simulink model "GNC2026"  (R2024b)
settings: Solver=ode4  StartTime=0.0  StopTime=tsim  FixedStep=baseRate
values from neighbouring files (symbols this model uses):
  a = 1    [Run_Initializer.m]    (also in UKFoptimization.m)
  a1 = 0.236940    (= 0.23694)    [DrawARM.m]    (also in Run_Initializer.m = 2)
  a2 = 0.281536    [DrawARM.m]    (also in Run_Initializer.m = 2)
  a3 = 0.0621    [DrawARM.m]    (also in Run_Initializer.m = 2)
  A_c = eye(3)    [Run_Initializer.m]
  alpha = diag([a1; a2; a3])    [Run_Initializer.m]    (also in overlapping_trajectories.m = alpha_values1(ii); plotTrajectory.m = alpha_values(ii); plotfig.m = alpha_values(ii))
  b = 2    [Run_Initializer.m]    (also in UKFoptimization.m)
  b0 = 0.230400    (= 0.2304)    [DrawARM.m]
  b1 = 0.078980    (= 0.07898)    [DrawARM.m]
  b2 = 0.070384    [DrawARM.m]
  b3 = 0.070685    [DrawARM.m]
  CVrate = 1/5    (= 0.2)    [Run_Initializer.m]
  dt = baseRate    [Run_Initializer.m]    (also in UKFoptimization.m = 0.05; rms_plots.m = median(diff(tA)))
  F_u = zeros(3,1)    [Run_Initializer.m]
  fNum = 1    [Run_Initializer.m]
  gamma = r - (excess + shrink + bracketwidth)    (= 0.05023)    [DrawSpacecraft.m]    (also in Run_Initializer.m = diag([g1; g2; g3]))
  Gamma1_el = 0.12    [Run_Initializer.m]
  Gamma1_sh = 0.005    [Run_Initializer.m]
  Gamma1_wr = 0.025    [Run_Initializer.m]
  Gamma2_el = 5    [Run_Initializer.m]
  Gamma2_sh = 5    [Run_Initializer.m]
  Gamma2_wr = 5    [Run_Initializer.m]
  Gamma3_el = 10    [Run_Initializer.m]
  Gamma3_sh = 40    [Run_Initializer.m]
  Gamma3_wr = 40    [Run_Initializer.m]
  Gamma4_el = 0.039    [Run_Initializer.m]
  Gamma4_sh = 0.015    [Run_Initializer.m]
  Gamma4_wr = 0.029    [Run_Initializer.m]
  Gamma5_el = 800    [Run_Initializer.m]
  Gamma5_sh = 800    [Run_Initializer.m]
  Gamma5_wr = 800    [Run_Initializer.m]
  Gamma6_el = 0.000001    (= 1e-06)    [Run_Initializer.m]
  Gamma6_sh = 0.005    [Run_Initializer.m]
  Gamma6_wr = 0.02    [Run_Initializer.m]
  k = 5    [Run_Initializer.m]    (also in UKFoptimization.m)
  Kd_elarm = 0.8    [Run_Initializer.m]
  Kd_sharm = 1.0    (= 1)    [Run_Initializer.m]
  Kd_wrarm = 0.6    [Run_Initializer.m]
  Kp_elarm = 1.2    [Run_Initializer.m]
  Kp_sharm = 1.5    [Run_Initializer.m]
  Kp_wrarm = 1.0    (= 1)    [Run_Initializer.m]
  Mc_inv = inv(M_c)    [Run_Initializer.m]
  Phi = 73.2749*pi/180    (= 1.27888826407)    [DrawARM.m]
  PWMFreq = 5    [Run_Initializer.m]
  R = [cos(theta) -sin(theta) ... (first row only)    [Run_Initializer.m]    (also in UKFoptimization.m = diag([rx, rx, rt]))
  sep1 = 0.60    (= 0.6)    [Run_Initializer.m]
  sep2 = 0.30    (= 0.3)    [Run_Initializer.m]
  sep3 = 0.30    (= 0.3)    [Run_Initializer.m]
  Tz_lim_elarm = .1    (= 0.1)    [Run_Initializer.m]
  Tz_lim_sharm = .1    (= 0.1)    [Run_Initializer.m]
  Tz_lim_wrarm = .1    (= 0.1)    [Run_Initializer.m]
  VISinLoop = 1    [Run_Initializer.m]
  X1_blk = 0.4    [Run_Initializer.m]
  X2_blk = 0.4    [Run_Initializer.m]
  X3_blk = 0.4    [Run_Initializer.m]
  Y1_blk = 0.4    [Run_Initializer.m]
  Y2_blk = 0.4    [Run_Initializer.m]
  Y3_blk = 0.4    [Run_Initializer.m]
undefined symbols (not defined in the file or in its folder): baseRate, dataRate, DiscIntNeverNeededParam, drop_states_ARM, drop_states_BLACK, drop_states_BLUE, drop_states_RED, F_red_X_nominal, F_red_Y_nominal, F_thrusters_BLACK, F_thrusters_BLUE, F_thrusters_RED, home_states_BLACK, home_states_BLUE, home_states_RED, IBLACK, IBLUE, IDIST, IEE, init_states_BLACK, init_states_BLUE, init_states_RED, IPROX, IRED, K_BLACK, K_BLUE, K_RED, Kd_tb, Kd_tblue, Kd_tr, Kd_xb, Kd_xblue, Kd_xr, Kd_yb, Kd_yblue, Kd_yr, Kp_tb, Kp_tblue, Kp_tr, Kp_xb, Kp_xblue, Kp_xr, Kp_yb, Kp_yblue, Kp_yr, mBLACK, mBLUE, mDIST, mEE, mPROX, mRED, Phase0_End, Phase1_End, Phase2_End, Phase3_End, Phase3_SubPhase1_End, Phase3_SubPhase2_End, Phase3_SubPhase3_End, Phase3_SubPhase4_End, Phase4_End ... (+10)
libraries: simulink x30, nvidiaSharedBlocks x20, MainLibrary x5, dspinverses x3, commrandsrc3 x1, nvidiaIMUSensorslib x1
(part 4 of 9)

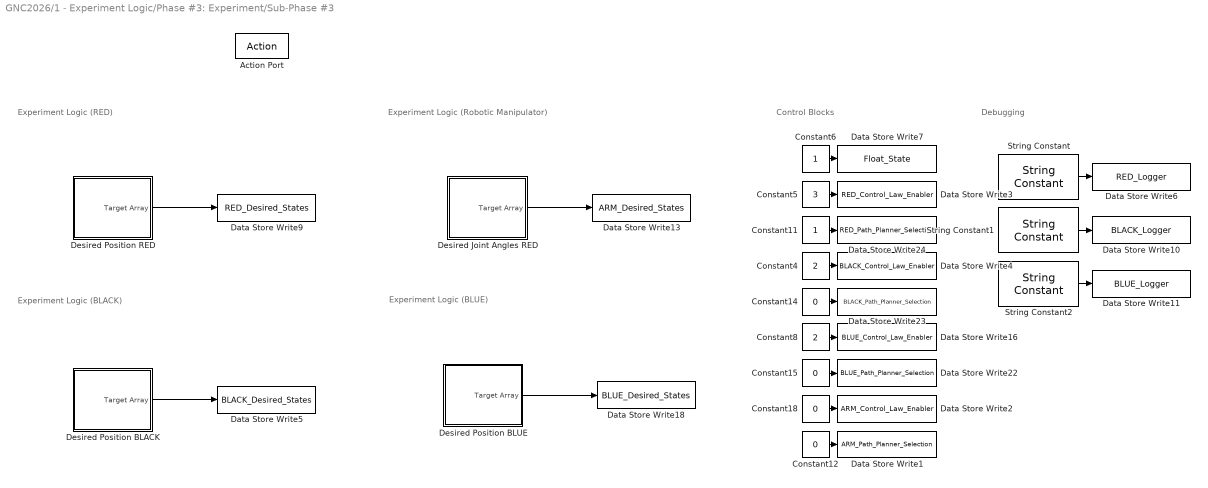
== system GNC2026/1 - Experiment Logic/Phase #3: Experiment/Sub-Phase #3  ==
  note: Experiment Logic (BLACK)
  note: Experiment Logic (Robotic Manipulator)
  note: Experiment Logic (BLUE)
  note: Experiment Logic (RED)
  note: Control Blocks
  note: Debugging
  Action Port : ActionPort  ActionPortLabel=elseif((u1 < u4 & u1 >= u3))
  Constant11 : Constant
  Constant{12,14..15,18} (4 alike) : Constant  Value=0
  Constant4 : Constant  Value=2
  Constant5 : Constant  Value=3
  Constant6 : Constant
  Constant8 : Constant  Value=2
  Data Store Write1 : DataStoreWrite  DataStoreName=ARM_Path_Planner_Selection  IndexOptions=Index vector (dialog)  Indices=1  OutputSizes=1
  Data Store Write10 : DataStoreWrite  DataStoreName=BLACK_Logger  IndexOptions=Index vector (dialog)  Indices=1  OutputSizes=1
  Data Store Write11 : DataStoreWrite  DataStoreName=BLUE_Logger  IndexOptions=Index vector (dialog)  Indices=1  OutputSizes=1
  Data Store Write13 : DataStoreWrite  DataStoreName=ARM_Desired_States  IndexOptions=Index vector (dialog)  Indices=1  OutputSizes=1
  Data Store Write16 : DataStoreWrite  DataStoreName=BLUE_Control_Law_Enabler  IndexOptions=Index vector (dialog)  Indices=1  OutputSizes=1
  Data Store Write18 : DataStoreWrite  DataStoreName=BLUE_Desired_States  IndexOptions=Index vector (dialog)  Indices=1  OutputSizes=1
  Data Store Write2 : DataStoreWrite  DataStoreName=ARM_Control_Law_Enabler  IndexOptions=Index vector (dialog)  Indices=1  OutputSizes=1
  Data Store Write22 : DataStoreWrite  DataStoreName=BLUE_Path_Planner_Selection  IndexOptions=Index vector (dialog)  Indices=1  OutputSizes=1
  Data Store Write23 : DataStoreWrite  DataStoreName=BLACK_Path_Planner_Selection  IndexOptions=Index vector (dialog)  Indices=1  OutputSizes=1
  Data Store Write24 : DataStoreWrite  DataStoreName=RED_Path_Planner_Selection  IndexOptions=Index vector (dialog)  Indices=1  OutputSizes=1
  Data Store Write3 : DataStoreWrite  DataStoreName=RED_Control_Law_Enabler  IndexOptions=Index vector (dialog)  Indices=1  OutputSizes=1
  Data Store Write4 : DataStoreWrite  DataStoreName=BLACK_Control_Law_Enabler  IndexOptions=Index vector (dialog)  Indices=1  OutputSizes=1
  Data Store Write5 : DataStoreWrite  DataStoreName=BLACK_Desired_States  IndexOptions=Index vector (dialog)  Indices=1  OutputSizes=1
  Data Store Write6 : DataStoreWrite  DataStoreName=RED_Logger  IndexOptions=Index vector (dialog)  Indices=1  OutputSizes=1
  Data Store Write7 : DataStoreWrite  DataStoreName=Float_State  IndexOptions=Index vector (dialog)  Indices=1  OutputSizes=1
  Data Store Write9 : DataStoreWrite  DataStoreName=RED_Desired_States  IndexOptions=Index vector (dialog)  Indices=1  OutputSizes=1
  Desired Joint Angles RED : Subsystem
  Desired Position BLACK : Subsystem
  Desired Position BLUE : Subsystem
  Desired Position RED : Subsystem
  String Constant : StringConstant  String="\"Chaser: Running Phase 3 Sub-Phase 3\""
  String Constant1 : StringConstant  String="\"Target: Running Phase 3 Sub-Phase 3\""
  String Constant2 : StringConstant  String="\"Obstacle: Running Phase 3 Sub-Phase 3\""
  wires:
  Desired Position RED/1(Target Array) -> Data Store Write9/1
  Desired Position BLACK/1(Target Array) -> Data Store Write5/1
  Desired Position BLUE/1(Target Array) -> Data Store Write18/1
  Desired Joint Angles RED/1(Target Array) -> Data Store Write13/1
  Constant12/1 -> Data Store Write1/1
  Constant18/1 -> Data Store Write2/1
  Constant6/1 -> Data Store Write7/1
  Constant15/1 -> Data Store Write22/1
  Constant14/1 -> Data Store Write23/1
  Constant5/1 -> Data Store Write3/1
  Constant11/1 -> Data Store Write24/1
  Constant8/1 -> Data Store Write16/1
  Constant4/1 -> Data Store Write4/1
  String Constant1/1 -> Data Store Write10/1
  String Constant/1 -> Data Store Write6/1
  String Constant2/1 -> Data Store Write11/1

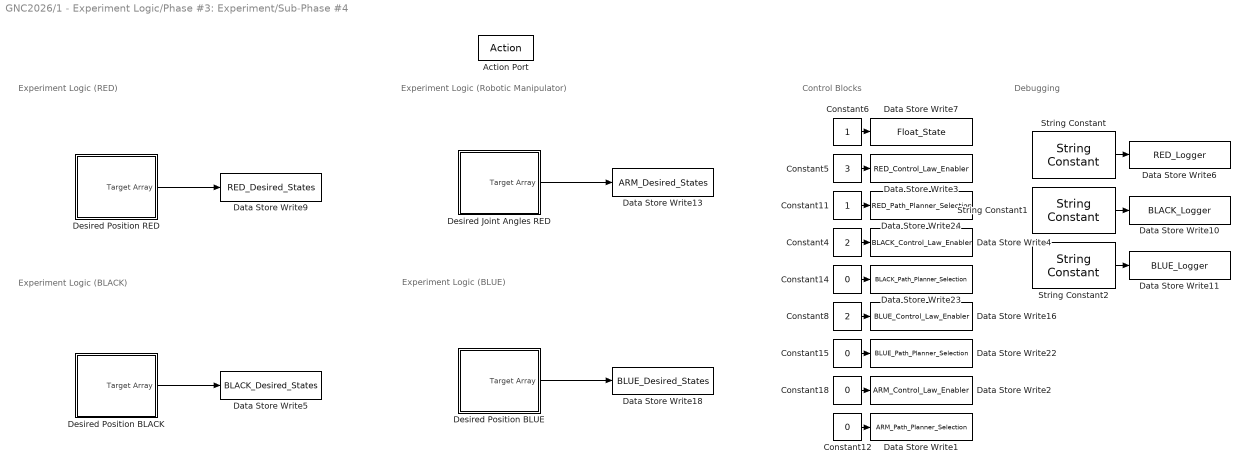
== system GNC2026/1 - Experiment Logic/Phase #3: Experiment/Sub-Phase #4 ==
  note: Experiment Logic (BLACK)
  note: Experiment Logic (Robotic Manipulator)
  note: Experiment Logic (BLUE)
  note: Experiment Logic (RED)
  note: Control Blocks
  note: Debugging
  Action Port : ActionPort  ActionPortLabel=elseif( (u1 < u5 & u1 >= u4))
  Constant11 : Constant
  Constant{12,14..15,18} (4 alike) : Constant  Value=0
  Constant4 : Constant  Value=2
  Constant5 : Constant  Value=3
  Constant6 : Constant
  Constant8 : Constant  Value=2
  Data Store Write1 : DataStoreWrite  DataStoreName=ARM_Path_Planner_Selection  IndexOptions=Index vector (dialog)  Indices=1  OutputSizes=1
  Data Store Write10 : DataStoreWrite  DataStoreName=BLACK_Logger  IndexOptions=Index vector (dialog)  Indices=1  OutputSizes=1
  Data Store Write11 : DataStoreWrite  DataStoreName=BLUE_Logger  IndexOptions=Index vector (dialog)  Indices=1  OutputSizes=1
  Data Store Write13 : DataStoreWrite  DataStoreName=ARM_Desired_States  IndexOptions=Index vector (dialog)  Indices=1  OutputSizes=1
  Data Store Write16 : DataStoreWrite  DataStoreName=BLUE_Control_Law_Enabler  IndexOptions=Index vector (dialog)  Indices=1  OutputSizes=1
  Data Store Write18 : DataStoreWrite  DataStoreName=BLUE_Desired_States  IndexOptions=Index vector (dialog)  Indices=1  OutputSizes=1
  Data Store Write2 : DataStoreWrite  DataStoreName=ARM_Control_Law_Enabler  IndexOptions=Index vector (dialog)  Indices=1  OutputSizes=1
  Data Store Write22 : DataStoreWrite  DataStoreName=BLUE_Path_Planner_Selection  IndexOptions=Index vector (dialog)  Indices=1  OutputSizes=1
  Data Store Write23 : DataStoreWrite  DataStoreName=BLACK_Path_Planner_Selection  IndexOptions=Index vector (dialog)  Indices=1  OutputSizes=1
  Data Store Write24 : DataStoreWrite  DataStoreName=RED_Path_Planner_Selection  IndexOptions=Index vector (dialog)  Indices=1  OutputSizes=1
  Data Store Write3 : DataStoreWrite  DataStoreName=RED_Control_Law_Enabler  IndexOptions=Index vector (dialog)  Indices=1  OutputSizes=1
  Data Store Write4 : DataStoreWrite  DataStoreName=BLACK_Control_Law_Enabler  IndexOptions=Index vector (dialog)  Indices=1  OutputSizes=1
  Data Store Write5 : DataStoreWrite  DataStoreName=BLACK_Desired_States  IndexOptions=Index vector (dialog)  Indices=1  OutputSizes=1
  Data Store Write6 : DataStoreWrite  DataStoreName=RED_Logger  IndexOptions=Index vector (dialog)  Indices=1  OutputSizes=1
  Data Store Write7 : DataStoreWrite  DataStoreName=Float_State  IndexOptions=Index vector (dialog)  Indices=1  OutputSizes=1
  Data Store Write9 : DataStoreWrite  DataStoreName=RED_Desired_States  IndexOptions=Index vector (dialog)  Indices=1  OutputSizes=1
  Desired Joint Angles RED : Subsystem
  Desired Position BLACK : Subsystem
  Desired Position BLUE : Subsystem
  Desired Position RED : Subsystem
  String Constant : StringConstant  String="\"Chaser: Running Phase 3 Sub-Phase 4\""
  String Constant1 : StringConstant  String="\"Target: Running Phase 3 Sub-Phase 4\""
  String Constant2 : StringConstant  String="\"Obstacle: Running Phase 3 Sub-Phase 4\""
  wires:
  Desired Position RED/1(Target Array) -> Data Store Write9/1
  Desired Position BLACK/1(Target Array) -> Data Store Write5/1
  Desired Position BLUE/1(Target Array) -> Data Store Write18/1
  Desired Joint Angles RED/1(Target Array) -> Data Store Write13/1
  Constant12/1 -> Data Store Write1/1
  Constant18/1 -> Data Store Write2/1
  Constant6/1 -> Data Store Write7/1
  Constant15/1 -> Data Store Write22/1
  Constant14/1 -> Data Store Write23/1
  Constant5/1 -> Data Store Write3/1
  Constant11/1 -> Data Store Write24/1
  Constant8/1 -> Data Store Write16/1
  Constant4/1 -> Data Store Write4/1
  String Constant1/1 -> Data Store Write10/1
  String Constant/1 -> Data Store Write6/1
  String Constant2/1 -> Data Store Write11/1

== system GNC2026/1 - Experiment Logic/Phase #4: Return Home/Desired Joint Angles RED ==
  Constant1 : Constant  Value=pi/2
  Constant2 : Constant  Value=0
  Constant3 : Constant  Value=pi/2
  Mux : Mux  Inputs=3
  Target Array : Outport
  wires:
  Mux/1 -> Target Array/1
  Constant3/1 -> Mux/1
  Constant1/1 -> Mux/2
  Constant2/1 -> Mux/3

== system GNC2026/1 - Experiment Logic/Phase #4: Return Home/Desired Position BLACK ==
  Desired States (BLACK) : Constant  Value=home_states_BLACK  SampleTime=-1
  Target Array : Outport
  wires:
  Desired States (BLACK)/1 -> Target Array/1

== system GNC2026/1 - Experiment Logic/Phase #4: Return Home/Desired Position BLUE ==
  Desired States (BLUE) : Constant  Value=home_states_BLUE  SampleTime=-1
  Target Array : Outport
  wires:
  Desired States (BLUE)/1 -> Target Array/1

== system GNC2026/1 - Experiment Logic/Phase #4: Return Home/Desired Position RED ==
  Constant2 : Constant  Value=home_states_RED
  Target Array : Outport
  wires:
  Constant2/1 -> Target Array/1

== system GNC2026/1 - Experiment Logic/Phase #5: Hold Home/Desired Joint Angles RED ==
  Constant1 : Constant  Value=pi/2
  Constant2 : Constant  Value=0
  Constant3 : Constant  Value=pi/2
  Mux : Mux  Inputs=3
  Target Array : Outport
  wires:
  Mux/1 -> Target Array/1
  Constant3/1 -> Mux/1
  Constant1/1 -> Mux/2
  Constant2/1 -> Mux/3

== system GNC2026/1 - Experiment Logic/Phase #5: Hold Home/Desired Position BLACK ==
  Desired States (BLACK) : Constant  Value=home_states_BLACK  SampleTime=-1
  Target Array : Outport
  wires:
  Desired States (BLACK)/1 -> Target Array/1

== system GNC2026/1 - Experiment Logic/Phase #5: Hold Home/Desired Position BLUE ==
  Desired States (BLUE) : Constant  Value=home_states_BLUE  SampleTime=-1
  Target Array : Outport
  wires:
  Desired States (BLUE)/1 -> Target Array/1

== system GNC2026/1 - Experiment Logic/Phase #5: Hold Home/Desired Position RED ==
  Constant2 : Constant  Value=home_states_RED
  Target Array : Outport
  wires:
  Constant2/1 -> Target Array/1

== system GNC2026/2 - Guidance/Custom PPL (ARM)/Desired Position ==
  Data Store Read : DataStoreRead  DataStoreName=ARM_Desired_States  IndexOptions=Index vector (dialog)  Indices=1  OutputSizes=1
  Position Array : Outport
  wires:
  Data Store Read/1 -> Position Array/1

== system GNC2026/2 - Guidance/Custom PPL (BLACK)/Desired Position ==
  BLACK_Px : DataStoreRead  DataStoreName=BLACK_Desired_States  IndexOptions=Index vector (dialog)  Indices=1  OutputSizes=1
  Position Array : Outport
  wires:
  BLACK_Px/1 -> Position Array/1

== system GNC2026/2 - Guidance/Custom PPL (BLUE)/Desired Position ==
  Data Store Read4 : DataStoreRead  DataStoreName=BLUE_Desired_States  IndexOptions=Index vector (dialog)  Indices=1  OutputSizes=1
  Position Array : Outport
  wires:
  Data Store Read4/1 -> Position Array/1

== system GNC2026/2 - Guidance/Custom PPL (RED)/Unwrap1 ==
  In1 : Inport
  Demux : Demux  Outputs=3
  Mux1 : Mux  Inputs=3
  Unwrap : Subsystem
  Unwrap1 : Subsystem  Commented=on
  Out1 : Outport
  wires:
  Demux/2 -> Mux1/2
  Demux/3 -> Unwrap/1(u)
  Demux/1 -> Mux1/1
  Unwrap/1(y) -> Mux1/3
  In1/1 -> Demux/1
  Mux1/1 -> Out1/1

== system GNC2026/2 - Guidance/Disable PPL (ARM)/Desired Position ==
  Data Store Read : DataStoreRead  DataStoreName=ARM_Desired_States  IndexOptions=Index vector (dialog)  Indices=1  OutputSizes=1
  Position Array : Outport
  wires:
  Data Store Read/1 -> Position Array/1

== system GNC2026/2 - Guidance/Disable PPL (BLACK)/Desired Position ==
  BLACK_Px : DataStoreRead  DataStoreName=BLACK_Desired_States  IndexOptions=Index vector (dialog)  Indices=1  OutputSizes=1
  Position Array : Outport
  wires:
  BLACK_Px/1 -> Position Array/1

== system GNC2026/2 - Guidance/Disable PPL (BLUE)/Desired Position ==
  Data Store Read4 : DataStoreRead  DataStoreName=BLUE_Desired_States  IndexOptions=Index vector (dialog)  Indices=1  OutputSizes=1
  Position Array : Outport
  wires:
  Data Store Read4/1 -> Position Array/1

== system GNC2026/2 - Guidance/Disable PPL (RED)/Desired Position ==
  RED_Px : DataStoreRead  DataStoreName=RED_Desired_States  IndexOptions=Index vector (dialog)  Indices=1  OutputSizes=1
  Position Array : Outport
  wires:
  RED_Px/1 -> Position Array/1

== system GNC2026/3 - Control/Custom Control (RED)/Unwrap ==
  In1 : Inport
  Demux : Demux  Outputs=3
  Mux1 : Mux  Inputs=3
  Mux2 : Mux  Inputs=2
  Reshape : Reshape  OutputDimensionality=Customize  OutputDimensions=[9,1]
  Selector1 : Selector  InputPortWidth=9  IndexOptions=Index vector (dialog)  Indices=[4 5 6 7 8 9]  OutputSizes=1
  Selector4 : Selector  InputPortWidth=9  IndexOptions=Index vector (dialog)  Indices=[1 2 3]  OutputSizes=1
  Unwrap : Subsystem
  Out1 : Outport
  wires:
  Demux/2 -> Mux1/2
  Demux/3 -> Unwrap/1(u)
  Demux/1 -> Mux1/1
  Unwrap/1(y) -> Mux1/3
  Selector4/1 -> Demux/1
  In1/1 -> Selector1/1, Selector4/1
  Selector1/1 -> Mux2/2
  Mux2/1 -> Reshape/1
  Mux1/1 -> Mux2/1
  Reshape/1 -> Out1/1

== system GNC2026/3 - Control/Custom Control (RED)/Unwrap1 ==
  In1 : Inport
  Delay : Delay  DelayLength=1  InitialCondition=init_states_RED(3)  InputProcessing=Columns as channels (frame based)
  Delay1 : Delay  DelayLength=1  InitialCondition=init_states_RED(3)  InputProcessing=Columns as channels (frame based)
  MATLAB Function : MATLAB Function  TreatAsAtomicUnit=on
  Out1 : Outport
  wires:
  MATLAB Function/1(y) -> Out1/1, Delay1/1
  In1/1 -> MATLAB Function/1(u)
  MATLAB Function/2(u_next) -> Delay/1
  Delay/1 -> MATLAB Function/2(u_pre)
  Delay1/1 -> MATLAB Function/3(y_pre)

== system GNC2026/3 - Control/Default LQR Control (BLACK)/Calculate Error ==
  Desired Attitude : Inport
  Measured Attitude : Inport  Port=2
  MATLAB Function : MATLAB Function  TreatAsAtomicUnit=on
  Attitude Error : Outport
  wires:
  MATLAB Function/1(Rz_error) -> Attitude Error/1
  Desired Attitude/1 -> MATLAB Function/1(Rz_path)
  Measured Attitude/1 -> MATLAB Function/2(Rz_measured)

== system GNC2026/3 - Control/Default LQR Control (BLUE)/Calculate Error ==
  Desired Attitude : Inport
  Measured Attitude : Inport  Port=2
  MATLAB Function : MATLAB Function  TreatAsAtomicUnit=on
  Attitude Error : Outport
  wires:
  MATLAB Function/1(Rz_error) -> Attitude Error/1
  Desired Attitude/1 -> MATLAB Function/1(Rz_path)
  Measured Attitude/1 -> MATLAB Function/2(Rz_measured)

== system GNC2026/3 - Control/Default LQR Control (RED)/Calculate Error ==
  Desired Attitude : Inport
  Measured Attitude : Inport  Port=2
  MATLAB Function : MATLAB Function  TreatAsAtomicUnit=on
  Attitude Error : Outport
  wires:
  MATLAB Function/1(Rz_error) -> Attitude Error/1
  Desired Attitude/1 -> MATLAB Function/1(Rz_path)
  Measured Attitude/1 -> MATLAB Function/2(Rz_measured)

== system GNC2026/3 - Control/Default PD (ARM)/Passthrough for Experiment ==
  q1_desired : Inport
  q2_desired : Inport  Port=2
  q3_desired : Inport  Port=3
  Action Port : ActionPort  ActionPortLabel=else
  q1_command : Outport
  q2_command : Outport  Port=2
  q3_command : Outport  Port=3
  wires:
  q3_desired/1 -> q3_command/1
  q1_desired/1 -> q1_command/1
  q2_desired/1 -> q2_command/1

== system GNC2026/3 - Control/Default PD (ARM)/Simulated Position Controller ==
  q1_desired : Inport
  q2_desired : Inport  Port=2
  q3_desired : Inport  Port=3
  Action Port : ActionPort  ActionPortLabel=if(u1 == 1)
  Custom Discrete PD (Elbow) : Subsystem
  Custom Discrete PD (Shoulder) : Subsystem
  Custom Discrete PD (Wrist) : Subsystem
  Data Store Read2 : DataStoreRead  DataStoreName=ARM_Measured_States  IndexOptions=Index vector (dialog)  Indices=1  OutputSizes=1
  Demux : Demux  Outputs=[1,1,1,3]
  Saturation : Saturate  UpperLimit=Tz_lim_sharm  LowerLimit=-Tz_lim_sharm
  Saturation1 : Saturate  UpperLimit=Tz_lim_elarm  LowerLimit=-Tz_lim_elarm
  Saturation3 : Saturate  UpperLimit=Tz_lim_wrarm  LowerLimit=-Tz_lim_wrarm
  Subtract2 : Sum  Inputs=+-
  Subtract3 : Sum  Inputs=+-
  Subtract4 : Sum  Inputs=+-
  Terminator : Terminator
  q1_command : Outport
  q2_command : Outport  Port=2
  q3_command : Outport  Port=3
  wires:
  Saturation3/1 -> q3_command/1
  Subtract4/1 -> Custom Discrete PD (Wrist)/1(ey)
  Custom Discrete PD (Shoulder)/1(Fx) -> Saturation/1
  Custom Discrete PD (Elbow)/1(Fy) -> Saturation1/1
  Saturation/1 -> q1_command/1
  Subtract2/1 -> Custom Discrete PD (Shoulder)/1(ex)
  Saturation1/1 -> q2_command/1
  Custom Discrete PD (Wrist)/1(Fy) -> Saturation3/1
  Subtract3/1 -> Custom Discrete PD (Elbow)/1(ey)
  Demux/1 -> Subtract2/2
  Demux/2 -> Subtract3/2
  Demux/3 -> Subtract4/2
  q1_desired/1 -> Subtract2/1
  q2_desired/1 -> Subtract3/1
  q3_desired/1 -> Subtract4/1
  Data Store Read2/1 -> Demux/1
  Demux/4 -> Terminator/1

== system GNC2026/3 - Control/Default PD Control (BLACK)/Calculate Error ==
  Desired Attitude : Inport
  Measured Attitude : Inport  Port=2
  MATLAB Function : MATLAB Function  TreatAsAtomicUnit=on
  Attitude Error : Outport
  wires:
  MATLAB Function/1(Rz_error) -> Attitude Error/1
  Desired Attitude/1 -> MATLAB Function/1(Rz_path)
  Measured Attitude/1 -> MATLAB Function/2(Rz_measured)

== system GNC2026/3 - Control/Default PD Control (BLUE)/Calculate Error ==
  Desired Attitude : Inport
  Measured Attitude : Inport  Port=2
  MATLAB Function : MATLAB Function  TreatAsAtomicUnit=on
  Attitude Error : Outport
  wires:
  MATLAB Function/1(Rz_error) -> Attitude Error/1
  Desired Attitude/1 -> MATLAB Function/1(Rz_path)
  Measured Attitude/1 -> MATLAB Function/2(Rz_measured)

== system GNC2026/3 - Control/Default PD Control (RED)/Calculate Error ==
  Desired Attitude : Inport
  Measured Attitude : Inport  Port=2
  MATLAB Function : MATLAB Function  TreatAsAtomicUnit=on
  Attitude Error : Outport
  wires:
  MATLAB Function/1(Rz_error) -> Attitude Error/1
  Desired Attitude/1 -> MATLAB Function/1(Rz_path)
  Measured Attitude/1 -> MATLAB Function/2(Rz_measured)

== system GNC2026/Navigation Filter/If Action Subsystem/EKF ==
  note: Extended Kalman Filter
  Action Port : ActionPort  ActionPortLabel=elseif( u1 == 3)
  Artificial VIS States : Subsystem  TreatAsAtomicUnit=on
  Camera to Inertial Frame : MATLAB Function  TreatAsAtomicUnit=on
  Constant : Constant  Value=VISinLoop
  Data Store Read : DataStoreRead  DataStoreName=RED_Measured_States  DataStoreElements=RED_Measured_States(1:3)  IndexOptions=Index vector (dialog)  Indices=1  OutputSizes=1
  Data Store Read1 : DataStoreRead  Commented=on  DataStoreName=BLACK_CV_States  IndexOptions=Index vector (dialog)  Indices=1  OutputSizes=1
  Data Store Write2 : DataStoreWrite  DataStoreName=filterConfidence  IndexOptions=Index vector (dialog)  Indices=1  OutputSizes=1
  EKF : MATLAB Function  TreatAsAtomicUnit=on
  Experimental VIS States : Subsystem  TreatAsAtomicUnit=on
  If : If  IfExpression=u1 == 0  ElseIfExpressions=u1 == 1  ShowElse=off
  Merge : Merge
  Mux : Mux  Inputs=2
  Scope : Scope
  Unwrap : Subsystem
  BLKest : Outport
  wires:
  EKF/1(pose) -> Mux/1
  Mux/1 -> BLKest/1
  EKF/2(velocity) -> Mux/2
  Camera to Inertial Frame/1(r_T_I) -> EKF/1(black_cv_pose), Scope/1
  Data Store Read/1 -> Unwrap/1(In1)
  Unwrap/1(Out1) -> Camera to Inertial Frame/1(r_C_I)
  Constant/1 -> If/1
  Experimental VIS States/1(Out1) -> Merge/2
  If/2 -> Experimental VIS States/Action
  Artificial VIS States/1(Out1) -> Merge/1
  If/1 -> Artificial VIS States/Action
  Merge/1 -> Camera to Inertial Frame/2(r_REL_C)
  EKF/3(confidence) -> Data Store Write2/1

== system GNC2026/Navigation Filter/If Action Subsystem/MEKF ==
  note: Multiplicative Extended Kalman Filter
  Action Port : ActionPort  ActionPortLabel=elseif(u1 == 2)
  Artificial VIS States : Subsystem  TreatAsAtomicUnit=on
  Camera to Inertial Frame : MATLAB Function  TreatAsAtomicUnit=on
  Constant : Constant  Value=VISinLoop
  Data Store Read : DataStoreRead  DataStoreName=RED_Measured_States  DataStoreElements=RED_Measured_States(1:3)  IndexOptions=Index vector (dialog)  Indices=1  OutputSizes=1
  Data Store Read1 : DataStoreRead  Commented=on  DataStoreName=BLACK_CV_States  IndexOptions=Index vector (dialog)  Indices=1  OutputSizes=1
  Data Store Write2 : DataStoreWrite  DataStoreName=filterConfidence  IndexOptions=Index vector (dialog)  Indices=1  OutputSizes=1
  Experimental VIS States : Subsystem  TreatAsAtomicUnit=on
  If : If  IfExpression=u1 == 0  ElseIfExpressions=u1 == 1  ShowElse=off
  MEKF : MATLAB Function  TreatAsAtomicUnit=on
  Merge : Merge
  Mux : Mux  Inputs=2
  Scope : Scope
  Unwrap : Subsystem
  BLKest : Outport
  wires:
  MEKF/1(pose) -> Mux/1
  Mux/1 -> BLKest/1
  MEKF/2(velocity) -> Mux/2
  Unwrap/1(Out1) -> Camera to Inertial Frame/1(r_C_I)
  Data Store Read/1 -> Unwrap/1(In1)
  Camera to Inertial Frame/1(r_T_I) -> MEKF/1(black_cv_pose)
  Constant/1 -> If/1
  Experimental VIS States/1(Out1) -> Merge/2
  If/2 -> Experimental VIS States/Action
  Artificial VIS States/1(Out1) -> Merge/1
  If/1 -> Artificial VIS States/Action
  Merge/1 -> Camera to Inertial Frame/2(r_REL_C)
  MEKF/3(confidence) -> Scope/1, Data Store Write2/1

== system GNC2026/Navigation Filter/If Action Subsystem/UKF ==
  note: Unscented Kalman Filter
  Action Port : ActionPort  ActionPortLabel=if(u1 == 1)
  Artificial VIS States : Subsystem  TreatAsAtomicUnit=on
  Camera to Inertial Frame : MATLAB Function  TreatAsAtomicUnit=on
  Constant : Constant  Value=VISinLoop
  Data Store Read2 : DataStoreRead  DataStoreName=isValid  IndexOptions=Index vector (dialog)  Indices=1  OutputSizes=1
  Data Store Read3 : DataStoreRead  DataStoreName=RED_Measured_States  DataStoreElements=RED_Measured_States(1:3)  IndexOptions=Index vector (dialog)  Indices=1  OutputSizes=1
  Data Store Write2 : DataStoreWrite  DataStoreName=filterConfidence  IndexOptions=Index vector (dialog)  Indices=1  OutputSizes=1
  Experimental VIS States : Subsystem  TreatAsAtomicUnit=on
  If : If  IfExpression=u1 == 0  ElseIfExpressions=u1 == 1  ShowElse=off
  Merge : Merge
  Scope1 : Scope
  Scope2 : Scope
  Unit Delay1 : UnitDelay  InitialCondition=zeros(6,1)  SampleTime=-1  HasFrameUpgradeWarning=on
  Unit Delay2 : UnitDelay  InitialCondition=diag([1, 1, 0.05, 1, 1, 0.05])  SampleTime=-1  HasFrameUpgradeWarning=on
  Unscented Kalman Filter : MATLAB Function  TreatAsAtomicUnit=on
  Unwrap : Subsystem
  BLKest : Outport
  wires:
  Unscented Kalman Filter/1(x_est) -> Unit Delay1/1, BLKest/1
  Unit Delay2/1 -> Unscented Kalman Filter/4(P_pre)
  Unit Delay1/1 -> Unscented Kalman Filter/1(x_pre)
  Unscented Kalman Filter/3(P_est) -> Unit Delay2/1
  Camera to Inertial Frame/1(r_T_I) -> Scope2/1, Unscented Kalman Filter/2(y)
  Data Store Read3/1 -> Unwrap/1(In1)
  Unwrap/1(Out1) -> Camera to Inertial Frame/1(r_C_I)
  Data Store Read2/1 -> Unscented Kalman Filter/3(isValid)
  Merge/1 -> Camera to Inertial Frame/2(r_REL_C)
  Unscented Kalman Filter/2(confidence) -> Data Store Write2/1, Scope1/1
  Constant/1 -> If/1
  If/2 -> Experimental VIS States/Action
  If/1 -> Artificial VIS States/Action
  Artificial VIS States/1(Out1) -> Merge/1
  Experimental VIS States/1(Out1) -> Merge/2

== system GNC2026/PhaseSpace Camera Code/Use Hardware to Obtain States/Receive and Process Phasespace Data ==
  Check for Sychronization (Updated) : Subsystem
  Demux2 : Demux  Outputs=[1,18]
  Mux : Mux  Inputs=2
  Receive PhaseSpace Data : nvidiaSharedBlocks/UDP Receive  localURL='0.0.0.0'  localPort=31534  remoteURL='0.0.0.0'  remotePort=-1  recvBufferSize=8192  signalDatatype=double  dims=19  isVarSize=off  showBlockingTime=off  blockingTime=0  sampletime=-1  blockPlatform=NVIDIA
  Reshape : Reshape  OutputDimensionality=Customize  OutputDimensions=[19,1]
  Terminator : Terminator
  PhaseSpace Data : Outport
  PhaseSpace Clock : Outport  Port=2
  wires:
  Reshape/1 -> Demux2/1
  Demux2/2 -> Mux/2
  Mux/1 -> PhaseSpace Data/1
  Receive PhaseSpace Data/2 -> Terminator/1
  Receive PhaseSpace Data/1 -> Reshape/1
  Demux2/1 -> PhaseSpace Clock/1
  Check for Sychronization (Updated)/1(ClockAdjusted) -> Mux/1

== system GNC2026/PhaseSpace Camera Code/Use Hardware to Obtain States/Store BLACK Data ==
  note: Store BLACK Positions and Velocities
  BLACK Data : Inport
  BLACK Velocities : Inport  Port=2
  PS Clock : Inport  Port=3
  Calculate True Time Step : Subsystem
      settings: PortSchema="{\"entries\":[{\"content\":{\"sides\":[{\"content\":{\"connectorIds\":[\"In1\"]},\"type\":\"ConnectorPlacement.EquallySpacedRectSide\",\"uuid\":\"62932c5c-f2a7-44c8-96b4-4a75bab3a126\"},{\"content\":{\"connectorIds\":[\"Out1\"],\"side\":\"RIGHT\"},\"type\":\"ConnectorPlacement.EquallySpacedRectSide\",\"uuid\":\"82b3b717-2171-4047-b0df-3cd41cf9dfc7\"},{\"content\":{\"side\":\"TOP\"},\"type\":\"ConnectorPlacement.EquallySpacedRectSide\",\"uuid\":\"a142272a-a0ff-4882-8a2d-4633b3c7e02f\"},{\"content\":{\"connectorIds\":[\"In2\"],\"side\":\"BOTTOM\"},\"type\":\"ConnectorPlacement.EquallySpacedRectSide\",\"uuid\":\"b1e1ff4c-66d6-488f-92fb-77f76780833b\"}]},\"type\":\"ConnectorPlacement.EquallySpacedConnector\",\"uuid\":\"98c51868-8a10-4b52-aae4-56f6042c65c4\"}],\"packageUris\":[\"http://schema.mathworks.com/mf0/Connector/R2020b\"],\"version\":\"1.0\"}"
  Convert BLACKVX from [mm] to [m] : Gain  Gain=1/1000
  Convert BLACKVY from [mm] to [m] : Gain  Gain=1/1000
  Convert BLAX from [mm] to [m] : Gain  Gain=1/1000
  Convert BLAY from [mm] to [m] : Gain  Gain=1/1000
  Demux : Demux  Outputs=3
  Demux2 : Demux  Outputs=3
  Demux3 : Demux  Outputs=3
  Mux{1..4} (4 alike) : Mux  Inputs=3
  RED_Px7 : DataStoreWrite  DataStoreName=BLACK_Measured_States  IndexOptions=Index vector (dialog)  Indices=1  OutputSizes=1
  Reshape : Reshape  OutputDimensionality=Column vector (2-D)
  Simulated Noise  (HARDWARE) : Subsystem
  Subsystem1 : Subsystem
  Subsystem2 : Subsystem
  Wrap : Subsystem
  wires:
  Demux3/1 -> Convert BLAX from [mm] to [m]/1
  Demux3/2 -> Convert BLAY from [mm] to [m]/1
  BLACK Data/1 -> Demux3/1
  Demux/3 -> Wrap/1(Unwrapped Angle)
  Reshape/1 -> Subsystem1/2(y)
  Demux/1 -> Mux1/1
  Convert BLAY from [mm] to [m]/1 -> Mux3/2
  Calculate True Time Step/1(dt_out) -> Subsystem2/1(dt), Subsystem1/1(dt)
  Mux3/1 -> Simulated Noise  (HARDWARE)/1(true states), Subsystem2/2(y), Demux/1, Calculate True Time Step/2(Data)
  Wrap/1(Wrapped Angle) -> Mux1/3
  Convert BLAX from [mm] to [m]/1 -> Mux3/1
  Mux2/1 -> RED_Px7/1
  Demux/2 -> Mux1/2
  Subsystem2/1(dy/dt) -> Reshape/1
  PS Clock/1 -> Calculate True Time Step/1(Time)
  Demux3/3 -> Mux3/3
  Subsystem1/1(dy/dt) -> Mux2/3
  BLACK Velocities/1 -> Demux2/1
  Demux2/3 -> Mux4/3
  Convert BLACKVX from [mm] to [m]/1 -> Mux4/1
  Convert BLACKVY from [mm] to [m]/1 -> Mux4/2
  Mux4/1 -> Mux2/2
  Demux2/2 -> Convert BLACKVY from [mm] to [m]/1
  Demux2/1 -> Convert BLACKVX from [mm] to [m]/1
  Mux1/1 -> Mux2/1

== system GNC2026/PhaseSpace Camera Code/Use Hardware to Obtain States/Store BLUE Data ==
  note: Store BLUE Positions and Velocities
  BLUE Data : Inport
  BLUE Velocities : Inport  Port=2
  PS Clock : Inport  Port=3
  Calculate True Time Step : Subsystem
      settings: PortSchema="{\"entries\":[{\"content\":{\"sides\":[{\"content\":{\"connectorIds\":[\"In1\"]},\"type\":\"ConnectorPlacement.EquallySpacedRectSide\",\"uuid\":\"62932c5c-f2a7-44c8-96b4-4a75bab3a126\"},{\"content\":{\"connectorIds\":[\"Out1\"],\"side\":\"RIGHT\"},\"type\":\"ConnectorPlacement.EquallySpacedRectSide\",\"uuid\":\"82b3b717-2171-4047-b0df-3cd41cf9dfc7\"},{\"content\":{\"side\":\"TOP\"},\"type\":\"ConnectorPlacement.EquallySpacedRectSide\",\"uuid\":\"a142272a-a0ff-4882-8a2d-4633b3c7e02f\"},{\"content\":{\"connectorIds\":[\"In2\"],\"side\":\"BOTTOM\"},\"type\":\"ConnectorPlacement.EquallySpacedRectSide\",\"uuid\":\"b1e1ff4c-66d6-488f-92fb-77f76780833b\"}]},\"type\":\"ConnectorPlacement.EquallySpacedConnector\",\"uuid\":\"98c51868-8a10-4b52-aae4-56f6042c65c4\"}],\"packageUris\":[\"http://schema.mathworks.com/mf0/Connector/R2020b\"],\"version\":\"1.0\"}"
  Convert BLUEVX from [mm] to [m] : Gain  Gain=1/1000
  Convert BLUEVY from [mm] to [m] : Gain  Gain=1/1000
  Convert BLUX from [mm] to [m] : Gain  Gain=1/1000
  Convert BLUY from [mm] to [m] : Gain  Gain=1/1000
  Demux : Demux  Outputs=3
  Demux2 : Demux  Outputs=3
  Demux5 : Demux  Outputs=3
  Mux{1..4} (4 alike) : Mux  Inputs=3
  RED_Px7 : DataStoreWrite  DataStoreName=BLUE_Measured_States  IndexOptions=Index vector (dialog)  Indices=1  OutputSizes=1
  Reshape : Reshape  OutputDimensionality=Column vector (2-D)
  Subsystem1 : Subsystem
  Subsystem2 : Subsystem
  Wrap : Subsystem
  wires:
  Demux5/2 -> Convert BLUY from [mm] to [m]/1
  Demux5/1 -> Convert BLUX from [mm] to [m]/1
  BLUE Data/1 -> Demux5/1
  Calculate True Time Step/1(dt_out) -> Subsystem2/1(dt), Subsystem1/1(dt)
  Demux/2 -> Mux1/2
  Demux/1 -> Mux1/1
  Subsystem2/1(dy/dt) -> Reshape/1
  Mux3/1 -> Subsystem2/2(y), Demux/1, Calculate True Time Step/2(Data)
  Demux/3 -> Wrap/1(Unwrapped Angle)
  Reshape/1 -> Subsystem1/2(y)
  Wrap/1(Wrapped Angle) -> Mux1/3
  Mux2/1 -> RED_Px7/1
  Convert BLUY from [mm] to [m]/1 -> Mux3/2
  Convert BLUX from [mm] to [m]/1 -> Mux3/1
  Demux5/3 -> Mux3/3
  PS Clock/1 -> Calculate True Time Step/1(Time)
  Mux1/1 -> Mux2/1
  Subsystem1/1(dy/dt) -> Mux2/3
  Demux2/1 -> Convert BLUEVX from [mm] to [m]/1
  Convert BLUEVY from [mm] to [m]/1 -> Mux4/2
  BLUE Velocities/1 -> Demux2/1
  Demux2/2 -> Convert BLUEVY from [mm] to [m]/1
  Mux4/1 -> Mux2/2
  Demux2/3 -> Mux4/3
  Convert BLUEVX from [mm] to [m]/1 -> Mux4/1

== system GNC2026/PhaseSpace Camera Code/Use Hardware to Obtain States/Store RED Data ==
  note: Store RED Position and Velocity Data
  RED Data : Inport
  RED Velocities : Inport  Port=2
  PS Clock : Inport  Port=3
  Calculate True Time Step : Subsystem
      settings: PortSchema="{\"entries\":[{\"content\":{\"sides\":[{\"content\":{\"connectorIds\":[\"In1\"]},\"type\":\"ConnectorPlacement.EquallySpacedRectSide\",\"uuid\":\"62932c5c-f2a7-44c8-96b4-4a75bab3a126\"},{\"content\":{\"connectorIds\":[\"Out1\"],\"side\":\"RIGHT\"},\"type\":\"ConnectorPlacement.EquallySpacedRectSide\",\"uuid\":\"82b3b717-2171-4047-b0df-3cd41cf9dfc7\"},{\"content\":{\"side\":\"TOP\"},\"type\":\"ConnectorPlacement.EquallySpacedRectSide\",\"uuid\":\"a142272a-a0ff-4882-8a2d-4633b3c7e02f\"},{\"content\":{\"connectorIds\":[\"In2\"],\"side\":\"BOTTOM\"},\"type\":\"ConnectorPlacement.EquallySpacedRectSide\",\"uuid\":\"b1e1ff4c-66d6-488f-92fb-77f76780833b\"}]},\"type\":\"ConnectorPlacement.EquallySpacedConnector\",\"uuid\":\"98c51868-8a10-4b52-aae4-56f6042c65c4\"}],\"packageUris\":[\"http://schema.mathworks.com/mf0/Connector/R2020b\"],\"version\":\"1.0\"}"
  Convert REDVX from [mm] to [m] : Gain  Gain=1/1000
  Convert REDVY from [mm] to [m] : Gain  Gain=1/1000
  Convert REDX from [mm] to [m] : Gain  Gain=1/1000
  Convert REDY from [mm] to [m] : Gain  Gain=1/1000
  Demux : Demux  Outputs=3
  Demux1 : Demux
  Demux2 : Demux  Outputs=3
  Mux{1..4} (4 alike) : Mux  Inputs=3
  RED_Px7 : DataStoreWrite  DataStoreName=RED_Measured_States  IndexOptions=Index vector (dialog)  Indices=1  OutputSizes=1
  Reshape : Reshape  OutputDimensionality=Column vector (2-D)
  Subsystem1 : Subsystem
  Subsystem2 : Subsystem
  Universal_Time : DataStoreWrite  DataStoreName=Univ_Time  IndexOptions=Index vector (dialog)  Indices=1  OutputSizes=1
  Wrap : Subsystem
  wires:
  Demux1/2 -> Convert REDX from [mm] to [m]/1
  Demux1/3 -> Convert REDY from [mm] to [m]/1
  RED Data/1 -> Demux1/1
  Demux1/4 -> Mux3/3
  Demux1/1 -> Universal_Time/1
  Mux2/1 -> RED_Px7/1
  Reshape/1 -> Subsystem1/2(y)
  Wrap/1(Wrapped Angle) -> Mux1/3
  Demux/3 -> Wrap/1(Unwrapped Angle)
  Demux/1 -> Mux1/1
  Subsystem2/1(dy/dt) -> Reshape/1
  Mux3/1 -> Subsystem2/2(y), Demux/1, Calculate True Time Step/2(Data)
  Demux/2 -> Mux1/2
  Convert REDX from [mm] to [m]/1 -> Mux3/1
  Convert REDY from [mm] to [m]/1 -> Mux3/2
  Calculate True Time Step/1(dt_out) -> Subsystem2/1(dt), Subsystem1/1(dt)
  Mux1/1 -> Mux2/1
  Subsystem1/1(dy/dt) -> Mux2/3
  Convert REDVX from [mm] to [m]/1 -> Mux4/1
  Convert REDVY from [mm] to [m]/1 -> Mux4/2
  Demux2/1 -> Convert REDVX from [mm] to [m]/1
  Demux2/2 -> Convert REDVY from [mm] to [m]/1
  Demux2/3 -> Mux4/3
  RED Velocities/1 -> Demux2/1
  Mux4/1 -> Mux2/2
  PS Clock/1 -> Calculate True Time Step/1(Time)

== system GNC2026/Receive CV Data/CV UDP/Reading isValid ==
  In1 : Inport
  Action Port : ActionPort  ActionPortLabel=if(u1 == 1)
  Data Store Write2 : DataStoreWrite  DataStoreName=isValid  IndexOptions=Index vector (dialog)  Indices=1  OutputSizes=1
  wires:
  In1/1 -> Data Store Write2/1

== system GNC2026/Simulate Plant Dynamics/BLACK Dynamics/Calculated & Store Measured States ==
  y : Inport
  dt : Inport  Port=2
  Demux : Demux  Outputs=3
  Measured States for BLACK : DataStoreWrite  DataStoreName=BLACK_Measured_States  IndexOptions=Index vector (dialog)  Indices=1  OutputSizes=1
  Mux1 : Mux  Inputs=3
  Mux2 : Mux  Inputs=3
  Reshape : Reshape  OutputDimensionality=Column vector (2-D)
  Subsystem1 : Subsystem
  Subsystem2 : Subsystem
  Wrap2 : Subsystem
  wires:
  Demux/1 -> Mux1/1
  Demux/2 -> Mux1/2
  Mux2/1 -> Measured States for BLACK/1
  Reshape/1 -> Subsystem1/2(y)
  Subsystem2/1(dy/dt) -> Mux2/2, Reshape/1
  y/1 -> Subsystem2/2(y), Demux/1
  Mux1/1 -> Mux2/1
  Subsystem1/1(dy/dt) -> Mux2/3
  dt/1 -> Subsystem1/1(dt), Subsystem2/1(dt)
  Demux/3 -> Wrap2/1(Unwrapped Angle)
  Wrap2/1(Wrapped Angle) -> Mux1/3

== system GNC2026/Simulate Plant Dynamics/BLACK Dynamics/Calculated & Store True States ==
  y : Inport
  Demux : Demux  Outputs=3
  Discrete Derivative : simulink/Discrete/Discrete Derivative  gainval=1.0  ICPrevScaledInput=0.0  OutMin=[]  OutMax=[]  OutDataType=fixdt(1, 16)  OutScaling=2^-10  DoSatur=off
  Discrete Derivative1 : simulink/Discrete/Discrete Derivative  gainval=1.0  ICPrevScaledInput=0.0  OutMin=[]  OutMax=[]  OutDataType=fixdt(1, 16)  OutScaling=2^-10  DoSatur=off
  Mux1 : Mux  Inputs=3
  Mux2 : Mux  Inputs=3
  True States for BLACK : DataStoreWrite  DataStoreName=BLACK_True_States  IndexOptions=Index vector (dialog)  Indices=1  OutputSizes=1
  Wrap1 : Subsystem
  wires:
  Demux/1 -> Mux1/1
  Demux/3 -> Wrap1/1(Unwrapped Angle)
  Demux/2 -> Mux1/2
  Mux2/1 -> True States for BLACK/1
  y/1 -> Discrete Derivative/1, Demux/1
  Discrete Derivative/1 -> Mux2/2, Discrete Derivative1/1
  Mux1/1 -> Mux2/1
  Discrete Derivative1/1 -> Mux2/3
  Wrap1/1(Wrapped Angle) -> Mux1/3

== system GNC2026/Simulate Plant Dynamics/BLACK Dynamics/Data @ Measurement Rate ==
  Data Input : Inport
  Calculate True Time Step : Subsystem
  Constant1 : Constant  Value=dataRate
  Constant2 : Constant  Value=0
  Data Store Read : DataStoreRead  DataStoreName=Univ_Time  IndexOptions=Index vector (dialog)  Indices=1  OutputSizes=1
  Delay : Delay  DelayLength=1
  Enabled Subsystem : Subsystem  TreatAsAtomicUnit=on
  Enabled Subsystem1 : Subsystem  TreatAsAtomicUnit=on
  Relational Operator1 : RelationalOperator  OutDataTypeStr=boolean  RndMeth=Simplest  InputSameDT=off
  Relational Operator2 : RelationalOperator  Operator===  OutDataTypeStr=boolean  RndMeth=Simplest  InputSameDT=off
  Subtract : Sum  Inputs=+-
  Data Held : Outport
  Time Step : Outport  Port=2
  wires:
  Data Input/1 -> Enabled Subsystem1/1(ThrustPer_Final)
  Subtract/1 -> Relational Operator2/1, Delay/1
  Relational Operator2/1 -> Enabled Subsystem1/Enable
  Relational Operator1/1 -> Enabled Subsystem/Enable
  Constant1/1 -> Calculate True Time Step/3(Rate), Relational Operator1/2
  Constant2/1 -> Relational Operator2/2
  Enabled Subsystem/1(Out1) -> Calculate True Time Step/2(Time), Subtract/2
  Delay/1 -> Relational Operator1/1
  Data Store Read/1 -> Enabled Subsystem/1(In1), Subtract/1
  Enabled Subsystem1/1(Out1) -> Calculate True Time Step/1(Data), Data Held/1
  Calculate True Time Step/1(dt_out) -> Time Step/1

== system GNC2026/Simulate Plant Dynamics/BLACK Dynamics/Dynamics Model for BLACK ==
  control_inputs : Inport
  Acceleration to Velocity : DiscreteIntegrator  IntegratorMethod=Integration: Backward Euler  SampleTime=-1  ICPrevOutput=DiscIntNeverNeededParam  ICPrevScaledInput=DiscIntNeverNeededParam
  MATLAB Function : MATLAB Function  TreatAsAtomicUnit=on
  Velocity to Position : DiscreteIntegrator  IntegratorMethod=Integration: Backward Euler  InitialCondition=drop_states_BLACK  SampleTime=-1  ICPrevOutput=DiscIntNeverNeededParam  ICPrevScaledInput=DiscIntNeverNeededParam
  states : Outport  VectorParamsAs1DForOutWhenUnconnected=off
  wires:
  control_inputs/1 -> MATLAB Function/1(control_inputs)
  MATLAB Function/1(x_ddot) -> Acceleration to Velocity/1
  Acceleration to Velocity/1 -> Velocity to Position/1
  Velocity to Position/1 -> states/1

== system GNC2026/Simulate Plant Dynamics/BLACK Dynamics/Simulated Noise  ==
  true states : Inport
  BLK CoM to LAR : MATLAB Function  TreatAsAtomicUnit=on
  CV Noise : MATLAB Function  TreatAsAtomicUnit=on
  Data Store Read : DataStoreRead  DataStoreName=BLACK_Exp_Noise  IndexOptions=Index vector (dialog)  Indices=1  OutputSizes=1
  Data Store Read3 : DataStoreRead  DataStoreName=RED_Measured_States  DataStoreElements=RED_Measured_States(1:3)  IndexOptions=Index vector (dialog)  Indices=1  OutputSizes=1
  Data Store Write : DataStoreWrite  DataStoreName=BLACK_CV_States  IndexOptions=Index vector (dialog)  Indices=1  OutputSizes=1
  Data Store Write2 : DataStoreWrite  DataStoreName=isValid  IndexOptions=Index vector (dialog)  Indices=1  OutputSizes=1
  Inertial to Camera Frame (SOFTWARE) : MATLAB Function  TreatAsAtomicUnit=on
  MATLAB Function1 : MATLAB Function  TreatAsAtomicUnit=on
  Sample and Hold : MATLAB Function  TreatAsAtomicUnit=on
  Scope{,2..4} (4 alike) : Scope
  Sum : Sum  Inputs=|++
  Unwrap : Subsystem
  wires:
  Data Store Read/1 -> Sum/2
  Sum/1 -> CV Noise/1(u)
  Data Store Read3/1 -> Unwrap/1(In1)
  CV Noise/1(y) -> Sample and Hold/1(u)
  Sample and Hold/1(y) -> Data Store Write/1, MATLAB Function1/1(LARstates_C_B)
  Unwrap/1(Out1) -> Inertial to Camera Frame (SOFTWARE)/1(r_C)
  MATLAB Function1/2(isValid) -> Scope/1, Data Store Write2/1
  Inertial to Camera Frame (SOFTWARE)/1(r_REL) -> Scope3/1, Sum/1
  true states/1 -> BLK CoM to LAR/1(r_T_I)
  BLK CoM to LAR/1(LARstates_I) -> Inertial to Camera Frame (SOFTWARE)/2(r_T), Scope4/1
  MATLAB Function1/1(data) -> Scope2/1

== system GNC2026/Simulate Plant Dynamics/BLUE Dynamics/BLUE  Dynamics Model ==
  control_inputs : Inport
  Acceleration to Velocity : DiscreteIntegrator  IntegratorMethod=Integration: Backward Euler  SampleTime=-1  ICPrevOutput=DiscIntNeverNeededParam  ICPrevScaledInput=DiscIntNeverNeededParam
  MATLAB Function : MATLAB Function  TreatAsAtomicUnit=on
  Velocity to Position : DiscreteIntegrator  IntegratorMethod=Integration: Backward Euler  InitialCondition=drop_states_BLUE  SampleTime=-1  ICPrevOutput=DiscIntNeverNeededParam  ICPrevScaledInput=DiscIntNeverNeededParam
  states : Outport  VectorParamsAs1DForOutWhenUnconnected=off
  wires:
  control_inputs/1 -> MATLAB Function/1(control_inputs)
  MATLAB Function/1(x_ddot) -> Acceleration to Velocity/1
  Acceleration to Velocity/1 -> Velocity to Position/1
  Velocity to Position/1 -> states/1

== system GNC2026/Simulate Plant Dynamics/BLUE Dynamics/Calculated & Store Measured States ==
  y : Inport
  dt : Inport  Port=2
  Demux : Demux  Outputs=3
  Measured States for BLUE : DataStoreWrite  DataStoreName=BLUE_Measured_States  IndexOptions=Index vector (dialog)  Indices=1  OutputSizes=1
  Mux1 : Mux  Inputs=3
  Mux2 : Mux  Inputs=3
  Reshape : Reshape  OutputDimensionality=Column vector (2-D)
  Subsystem1 : Subsystem
  Subsystem2 : Subsystem
  Wrap : Subsystem
  wires:
  Demux/1 -> Mux1/1
  Wrap/1(Wrapped Angle) -> Mux1/3
  Demux/3 -> Wrap/1(Unwrapped Angle)
  Demux/2 -> Mux1/2
  Mux2/1 -> Measured States for BLUE/1
  Reshape/1 -> Subsystem1/2(y)
  Subsystem2/1(dy/dt) -> Mux2/2, Reshape/1
  y/1 -> Subsystem2/2(y), Demux/1
  dt/1 -> Subsystem1/1(dt), Subsystem2/1(dt)
  Subsystem1/1(dy/dt) -> Mux2/3
  Mux1/1 -> Mux2/1

== system GNC2026/Simulate Plant Dynamics/BLUE Dynamics/Calculated & Store True States ==
  y : Inport
  Demux : Demux  Outputs=3
  Discrete Derivative : simulink/Discrete/Discrete Derivative  gainval=1.0  ICPrevScaledInput=0.0  OutMin=[]  OutMax=[]  OutDataType=fixdt(1, 16)  OutScaling=2^-10  DoSatur=off
  Discrete Derivative1 : simulink/Discrete/Discrete Derivative  gainval=1.0  ICPrevScaledInput=0.0  OutMin=[]  OutMax=[]  OutDataType=fixdt(1, 16)  OutScaling=2^-10  DoSatur=off
  Mux1 : Mux  Inputs=3
  Mux2 : Mux  Inputs=3
  True States for BLUE : DataStoreWrite  DataStoreName=BLUE_True_States  IndexOptions=Index vector (dialog)  Indices=1  OutputSizes=1
  Wrap : Subsystem
  wires:
  Demux/1 -> Mux1/1
  Wrap/1(Wrapped Angle) -> Mux1/3
  Demux/3 -> Wrap/1(Unwrapped Angle)
  Demux/2 -> Mux1/2
  Mux2/1 -> True States for BLUE/1
  Mux1/1 -> Mux2/1
  y/1 -> Discrete Derivative/1, Demux/1
  Discrete Derivative/1 -> Discrete Derivative1/1, Mux2/2
  Discrete Derivative1/1 -> Mux2/3

== system GNC2026/Simulate Plant Dynamics/BLUE Dynamics/Data @ Measurement Rate ==
  Data Input : Inport
  Calculate True Time Step : Subsystem
  Constant1 : Constant  Value=dataRate
  Constant2 : Constant  Value=0
  Data Store Read : DataStoreRead  DataStoreName=Univ_Time  IndexOptions=Index vector (dialog)  Indices=1  OutputSizes=1
  Delay : Delay  DelayLength=1
  Enabled Subsystem : Subsystem  TreatAsAtomicUnit=on
  Enabled Subsystem1 : Subsystem  TreatAsAtomicUnit=on
  Relational Operator1 : RelationalOperator  OutDataTypeStr=boolean  RndMeth=Simplest  InputSameDT=off
  Relational Operator2 : RelationalOperator  Operator===  OutDataTypeStr=boolean  RndMeth=Simplest  InputSameDT=off
  Subtract : Sum  Inputs=+-
  Data Held : Outport
  Time Step : Outport  Port=2
  wires:
  Data Input/1 -> Enabled Subsystem1/1(ThrustPer_Final)
  Subtract/1 -> Relational Operator2/1, Delay/1
  Relational Operator2/1 -> Enabled Subsystem1/Enable
  Relational Operator1/1 -> Enabled Subsystem/Enable
  Constant1/1 -> Calculate True Time Step/3(Rate), Relational Operator1/2
  Constant2/1 -> Relational Operator2/2
  Enabled Subsystem/1(Out1) -> Calculate True Time Step/2(Time), Subtract/2
  Delay/1 -> Relational Operator1/1
  Data Store Read/1 -> Enabled Subsystem/1(In1), Subtract/1
  Enabled Subsystem1/1(Out1) -> Calculate True Time Step/1(Data), Data Held/1
  Calculate True Time Step/1(dt_out) -> Time Step/1

== system GNC2026/Simulate Plant Dynamics/RED and ARM Dynamics/RED + ARM ==
  Action Port : ActionPort  ActionPortLabel=if(u1 == 4 | u1 == 5 | u1 == 10 | u1 == 11)
  Acceleration to Velocity : DiscreteIntegrator  IntegratorMethod=Integration: Backward Euler  InitialCondition=[0;0;0;0;0;0]  SampleTime=-1  ICPrevOutput=DiscIntNeverNeededParam  ICPrevScaledInput=DiscIntNeverNeededParam
  Add Noise : RandomNumber  Variance=1e-9  SampleTime=baseRate
  Calculated & Store Measured States : Subsystem
  Calculated & Store True States : Subsystem
  Coriolis Function1 : MATLAB Function  TreatAsAtomicUnit=on
  Data @ Measurement Rate : Subsystem
  Data Store Read3 : DataStoreRead  DataStoreName=ARM_Controls  IndexOptions=Index vector (dialog)  Indices=1  OutputSizes=1
  Delay : Delay  DelayLength=1
  Demux : Demux  Outputs=[1,1,10]
  Dynamics Model : MATLAB Function  TreatAsAtomicUnit=on
  Exceeded Table Limits : Subsystem
  Inertia Function 1 : MATLAB Function  TreatAsAtomicUnit=on
  Mux : Mux  Inputs=2
  Mux2 : Mux  Inputs=2
  Saturated Control Commands for RED : DataStoreRead  DataStoreName=RED_Saturated_Controls  IndexOptions=Index vector (dialog)  Indices=1  OutputSizes=1
  Stop Simulation : Stop
  Sum : Sum  Inputs=++|
  Terminator : Terminator
  Velocity to Position : DiscreteIntegrator  IntegratorMethod=Integration: Backward Euler  InitialCondition=[drop_states_RED,drop_states_ARM]  SampleTime=-1  ICPrevOutput=DiscIntNeverNeededParam  ICPrevScaledInput=DiscIntNeverNeededParam
  wires:
  Mux2/1 -> Dynamics Model/4(u)
  Data Store Read3/1 -> Mux2/2
  Dynamics Model/1(q_dot) -> Velocity to Position/1
  Coriolis Function1/1(CoriolisS) -> Dynamics Model/3(CoriolisS)
  Delay/1 -> Coriolis Function1/1(x), Inertia Function 1/1(x), Dynamics Model/1(x)
  Inertia Function 1/1(InertiaS) -> Dynamics Model/2(InertiaS)
  Saturated Control Commands for RED/1 -> Mux2/1
  Data @ Measurement Rate/2(Time Step) -> Calculated & Store Measured States/2(dt)
  Mux/1 -> Demux/1, Delay/1
  Dynamics Model/2(q_ddot) -> Acceleration to Velocity/1
  Acceleration to Velocity/1 -> Mux/2
  Demux/1 -> Exceeded Table Limits/1(X)
  Exceeded Table Limits/1(Stop) -> Stop Simulation/1
  Demux/2 -> Exceeded Table Limits/2(Y)
  Demux/3 -> Terminator/1
  Add Noise/1 -> Sum/1
  Velocity to Position/1 -> Sum/2, Calculated & Store True States/1(y), Mux/1
  Sum/1 -> Data @ Measurement Rate/1(Data Input)
  Data @ Measurement Rate/1(Data Held) -> Calculated & Store Measured States/1(y)
